simulink model "model"  (R2024a)
settings: Solver=FixedStepDiscrete  StartTime=0.0  StopTime=inf  FixedStep=0.01  RelTol=1e-3
libraries: simulink x1, spsMonostableLib x1
settings Model: Creator=Gabriel  LastModifiedBy=Gabriel

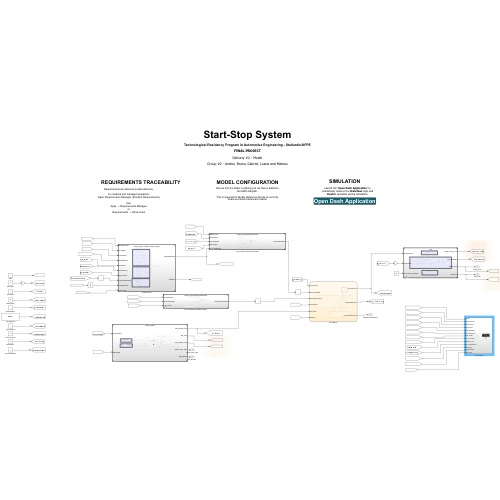
[thumbnail: Simulink's stored preview of the top-level diagram]
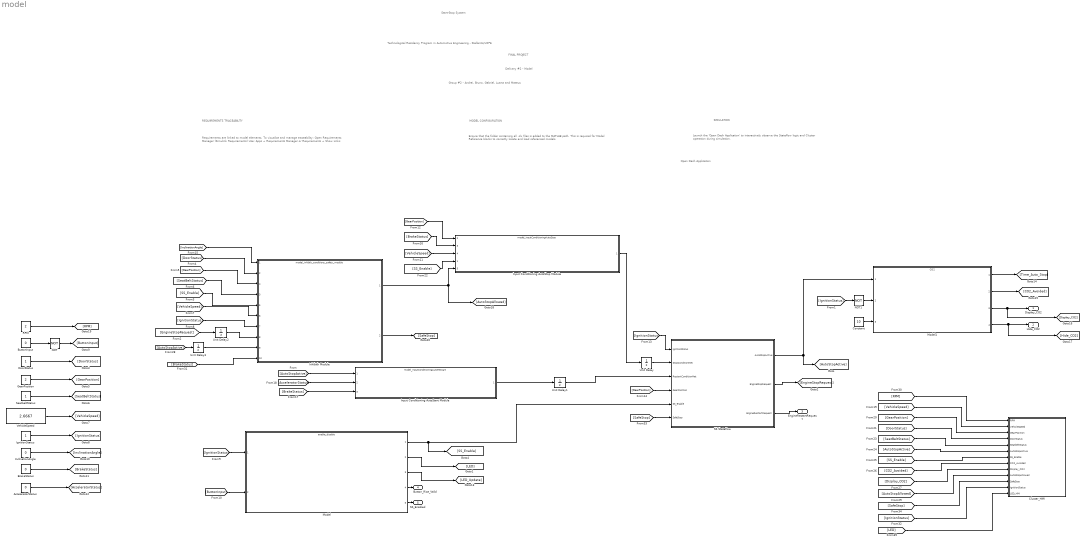
== system model ==
  note: Open Dash Application
  note: Technological Residency Program in Automotive Engineering - Stellantis/UFPE
  note: Start-Stop System
  note: FINAL PROJECT
  note: Group #2 - Andrei, Bruno, Gabriel, Luana and Mateus
  note: Delivery #2 - Model
  note: SIMULATION
  note: Launch the 'Open Dash Application' to interactively observe the Stateflow logic and Cluster operation during simulation.
  note: REQUIREMENTS TRACEABILITY
  note: Requirements are linked to model elements.
      |
      | To visualize and manage traceability:
      | Open Requirements Manager (Simulink Requirements)
      |
      | Use:
      | Apps → Requirements Manager
      | or
      | Requirements → Show Links
  note: Ensure that the folder containing all .slx files is added to the MATLAB path.
      |
      | This is required for Model Reference blocks to correctly locate and load referenced models.
  note: MODEL CONFIGURATION
  AcceleratorStatus : Constant  Value=0  OutDataTypeStr=boolean
  BrakeStatus : Constant  Value=0  OutDataTypeStr=boolean
  ButtonInput : Constant  Value=0  OutDataTypeStr=boolean
  Cluster_HMI : Subsystem
  Constant : Constant  Value=10
  DoorStatus : Constant  OutDataTypeStr=boolean
  GearPosition : Constant  Value=2
  IgnitionStatus : Constant  OutDataTypeStr=boolean
  InclinationAngle : Constant  Value=0
  Inhibith Module : ModelReference  ModelNameDialog=model_inhibth_conditions_safety_module.slx  SimulationMode=Normal  ModelReferenceVersion=1.14
      settings: PortSchema="{\"entries\":[{\"content\":{\"sides\":[{\"content\":{\"connectorIds\":[\"In1\",\"In2\",\"In4\",\"In3\",\"In5\",\"In6\",\"In7\",\"In8\",\"In9\",\"In10\"]},\"type\":\"ConnectorPlacement.EquallySpacedRectSide\",\"uuid\":\"a512ff0f-461c-49d9-bc5f-4a44ea731fcd\"},{\"content\":{\"connectorIds\":[\"Out1\",\"Out2\"],\"side\":\"RIGHT\"},\"type\":\"ConnectorPlacement.EquallySpacedRectSide\",\"uuid\":\"dd21159c-a948-4930-9666-9ab055a1217b\"},{\"content\":{\"side\":\"TOP\"},\"type\":\"ConnectorPlacement.EquallySpacedRectSide\",\"uuid\":\"5fbace01-0719-444d-b3d5-e5ff8fee5818\"}]},\"type\":\"ConnectorPlacement.EquallySpacedConnector\",\"uuid\":\"8aa1a26c-b679-4000-86cf-02a9aefd3465\"}],\"packageUris\":[\"http://schema.mathworks.com/mf0/Connector/R2020b\"],\"version\":\"1.0\"}"
  Input Conditioning AutoStart Module : ModelReference  ModelNameDialog=model_InputConditioningAutoRestart.slx  SimulationMode=Normal  ModelReferenceVersion=1.4
  Input Conditioning AutoStop Module : ModelReference  ModelNameDialog=model_InputConditioningAutoStop.slx  SimulationMode=Normal  ModelReferenceVersion=1.3
      settings: PortSchema="{\"entries\":[{\"content\":{\"sides\":[{\"content\":{\"connectorIds\":[\"In2\",\"In3\",\"In4\",\"In1\",\"In5\"]},\"type\":\"ConnectorPlacement.EquallySpacedRectSide\",\"uuid\":\"29c3241d-e620-43bc-b743-f10bc23ddf60\"},{\"content\":{\"connectorIds\":[\"Out1\"],\"side\":\"RIGHT\"},\"type\":\"ConnectorPlacement.EquallySpacedRectSide\",\"uuid\":\"375d0eb8-ed3e-4526-97ff-5015cdbb11d3\"},{\"content\":{\"side\":\"TOP\"},\"type\":\"ConnectorPlacement.EquallySpacedRectSide\",\"uuid\":\"7b1c3b74-98cc-495e-b24f-b127ed442c80\"}]},\"type\":\"ConnectorPlacement.EquallySpacedConnector\",\"uuid\":\"61a58fc7-57e7-4afa-ac3e-93f97ba24758\"}],\"packageUris\":[\"http://schema.mathworks.com/mf0/Connector/R2020b\"],\"version\":\"1.0\"}"
  Model : ModelReference  ModelNameDialog=enable_disable.slx  SimulationMode=Normal  ModelReferenceVersion=1.8
  Model1 : ModelReference  ModelNameDialog=CO2.slx  SimulationMode=Normal  ModelReferenceVersion=1.5
  NOT : Logic  Operator=NOT  IconShape=distinctive  AllPortsSameDT=off  OutDataTypeStr=boolean
  NOT1 : Logic  Operator=NOT  IconShape=distinctive  AllPortsSameDT=off  OutDataTypeStr=boolean
  RPM : Constant  Value=2  OutDataTypeStr=int8
  SS Stateflow : Stateflow chart  TreatAsAtomicUnit=on
  SeatbeltStatus : Constant  OutDataTypeStr=boolean
  Unit Delay : UnitDelay  SampleTime=-1  HasFrameUpgradeWarning=on
  Unit Delay1 : UnitDelay  SampleTime=-1  HasFrameUpgradeWarning=on
  Unit Delay2 : UnitDelay  SampleTime=0.1  HasFrameUpgradeWarning=on
  Unit Delay3 : UnitDelay  SampleTime=0.1  HasFrameUpgradeWarning=on
  VehicleSpeed : Constant  Value=2.6667
  Display_CO2 : Outport
  Hide_CO2 : Outport  Port=2
  EngineRestartRequest : Outport  Port=3
  Button_Rise_Valid : Outport  Port=4
  SS_Enabled : Outport  Port=5
  wires:
  DoorStatus/1 -> [DoorStatus]
  GearPosition/1 -> [GearPosition]
  SeatbeltStatus/1 -> [SeatBeltStatus]
  VehicleSpeed/1 -> [VehicleSpeed]
  IgnitionStatus/1 -> [IgnitionStatus]
  ButtonInput/1 -> NOT/1
  NOT/1 -> [ButtonInput]
  InclinationAngle/1 -> [InclinationAngle]
  BrakeStatus/1 -> [BrakeStatus]
  AcceleratorStatus/1 -> [AcceleratorStatus]
  Input Conditioning AutoStop Module/1 -> Unit Delay/1
  [GearPosition] -> Inhibith Module/4
  NOT1/1 -> Model1/2
  Model1/1 -> [Time_Auto_Stop]
  SS Stateflow/3(EngineRestartRequest) -> EngineRestartRequest/1
  [BrakeStatus] -> Input Conditioning AutoStart Module/3
  [VehicleSpeed] -> Input Conditioning AutoStop Module/4
  Model1/4 -> [Hide_CO2], Hide_CO2/1
  [GearPosition] -> Input Conditioning AutoStop Module/2
  Model1/3 -> [Display_CO2], Display_CO2/1
  [SS_Enable] -> Input Conditioning AutoStop Module/1
  Model/3 -> [LED_Update]
  Input Conditioning AutoStart Module/1 -> Unit Delay1/1
  Constant/1 -> Model1/3
  [InclinationAngle] -> Inhibith Module/1
  [IgnitionStatus] -> NOT1/1
  [IgnitionStatus] -> Model/1
  Model1/2 -> [CO2_Avoided]
  [GearPosition] -> SS Stateflow/4(GearPosition)
  Model/2 -> [LED]
  [ButtonInput] -> Model/2
  SS Stateflow/2(EngineStopRequest) -> [EngineStopRequest]
  [SeatBeltStatus] -> Inhibith Module/3
  [EngineStopRequest] -> Unit Delay2/1
  SS Stateflow/1(AutoStopActive) -> Model1/1, [AutoStopActive]
  Unit Delay1/1 -> SS Stateflow/3(RestartConditionMet)
  [IgnitionStatus] -> SS Stateflow/1(IgnitionStatus)
  Model/4 -> Button_Rise_Valid/1
  Inhibith Module/1 -> Input Conditioning AutoStop Module/5, [AutoStopAllowed]
  [VehicleSpeed] -> Inhibith Module/6
  [AcceleratorStatus] -> Input Conditioning AutoStart Module/2
  Unit Delay/1 -> SS Stateflow/2(StopConditionMet)
  [BrakeStatus] -> Input Conditioning AutoStop Module/3
  [DoorStatus] -> Inhibith Module/2
  [AutoStopActive] -> Input Conditioning AutoStart Module/1
  Model/5 -> SS_Enabled/1
  [SS_Enable] -> Inhibith Module/5
  [IgnitionStatus] -> Inhibith Module/7
  [VehicleSpeed] -> Cluster_HMI/2(VehicleSpeed)
  [GearPosition] -> Cluster_HMI/3(GearPosition)
  [DoorStatus] -> Cluster_HMI/4(DoorStatus)
  [SeatBeltStatus] -> Cluster_HMI/5(SeatbeltStatus)
  [AutoStopActive] -> Cluster_HMI/6(AutoStopActive)
  [CO2_Avoided] -> Cluster_HMI/8(CO2_Avoided)
  [Display_CO2] -> Cluster_HMI/9(Display_CO2)
  Model/1 -> [SS_Enable], SS Stateflow/5(SS_Enable)
  [SS_Enable] -> Cluster_HMI/7(SS_Enable)
  [AutoStopAllowed] -> Cluster_HMI/10(AutoStopAllowed)
  [RPM] -> Cluster_HMI/1(RPM)
  RPM/1 -> [RPM]
  [AutoStopActive] -> Unit Delay3/1
  [BrakeStatus] -> Inhibith Module/10
  Inhibith Module/2 -> [SafeStop]
  [SafeStop] -> SS Stateflow/6(SafeStop)
  [SafeStop] -> Cluster_HMI/11(SafeStop)
  Unit Delay2/1 -> Inhibith Module/8
  Unit Delay3/1 -> Inhibith Module/9
  [IgnitionStatus] -> Cluster_HMI/12(IgnitionStatus)
  [LED] -> Cluster_HMI/13(LED_HMI)

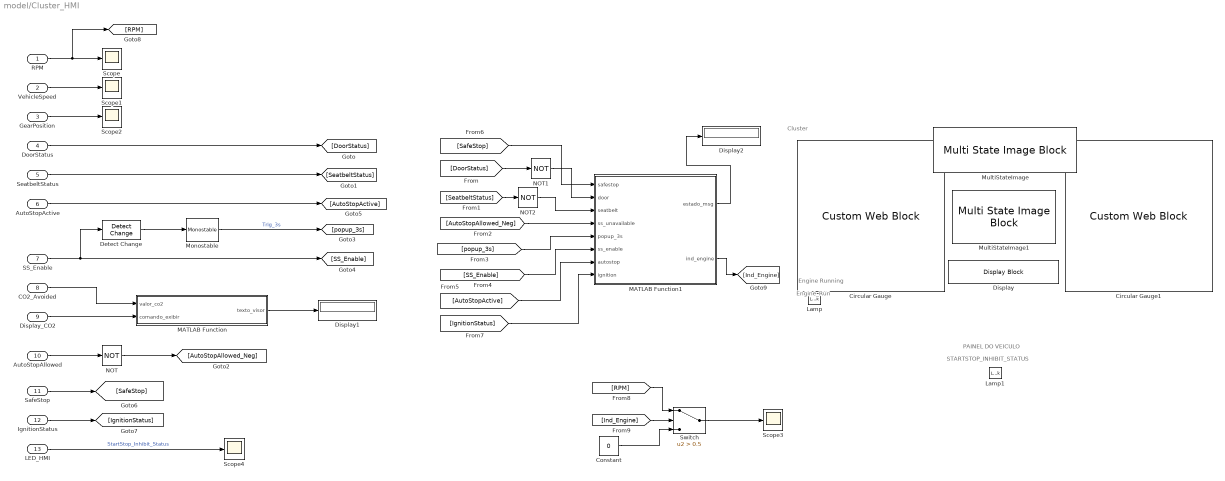
== system model/Cluster_HMI ==
  note: Engine_Run
  note: Engine Running
  note: Cluster
  note: PAINEL DO VEICULO
  note: STARTSTOP_INHIBIT_STATUS
  RPM : Inport
  VehicleSpeed : Inport  Port=2
  GearPosition : Inport  Port=3
  DoorStatus : Inport  Port=4
  SeatbeltStatus : Inport  Port=5
  AutoStopActive : Inport  Port=6
  SS_Enable : Inport  Port=7
  CO2_Avoided : Inport  Port=8
  Display_CO2 : Inport  Port=9
  AutoStopAllowed : Inport  Port=10
  SafeStop : Inport  Port=11
  IgnitionStatus : Inport  Port=12
  LED_HMI : Inport  Port=13
  Circular Gauge : CustomWebBlock  LabelPosition=Hide  ShowInitialText=on  Configuration="{\"components\":[{\"name\":\"CircularScaleComponent\",\"settings\":{\"bounds\":{\"max\":200,\"min\":0,\"tickInterval\":20},\"direction\":\"cw\",\"flipLimits\":0,\"innerRadius\":0.75,\"internalTickHeightScaleFactor\":1,\"labelColor\":[255,255,200],\"labelFont\":{\"font\":\"Arial\",\"fontSize\":12},\"labelRadius\":0.528,\"labelTransparency\":1,\"minorTickHeightScaleFactor\":0.2,\"needleImage\":{\"size\":[200,50],\"src\":\"data:image\\/svg+xml;base64,PD94bWwgdmVyc2lvbj0iMS4wIiBlbmNvZGluZz0idXRmLTgiPz4KPCEtLSBHZW5lcmF0b3I6IEFkb2JlIElsbHVzdHJhdG9yIDI0LjEuMiwgU1ZHIEV4cG9ydCBQbHVnLUluIC4gU1ZHIFZlcnNpb246IDYuMDAgQnVpbGQgMCkgIC0tPgo8c3ZnIHZlcnNpb249IjEuMSIgaWQ9IkxheWVyXzEiIHhtbG5zPSJodHRwOi8vd3d3LnczLm9yZy8yMDAwL3N2ZyIgeG1sbnM6eGxpbms9Imh0dHA6Ly93d3cudzMub3JnLzE5OTkveGxpbmsiIHg9IjBweCIgeT0iMHB4IgoJIHZpZXdCb3g9IjAgMCAyMDAgNTAiIHN0eWxlPSJlbmFibGUtYmFja2dyb3VuZDpuZXcgMCAwIDIwMCA1MDsiIHhtbDpzcGFjZT0icHJlc2VydmUiPgo8c3R5bGUgdHlwZT0idGV4dC9jc3MiPgoJLnN0MHtmaWxsOiNFQzIxMjc7fQo8L3N0eWxlPgo8cGF0aCBjbGFzcz0ic3QwIiBkPSJNMTYyLjgsMTMuN0MxNjksNC40LDE4MS43LDEuOSwxOTEsOC4xczExLjgsMTguOSw1LjYsMjguMnMtMTguOSwxMS44LTI4LjIsNS42bDAsMAoJQzE1OS4xLDM1LjYsMTU2LjYsMjMsMTYyLjgsMTMuN0wxNjIuOCwxMy43eiBNMTY1LjgsMTUuOGMtNS4xLDcuNi0zLjEsMTcuOSw0LjYsMjNjNy42LDUuMSwxNy45LDMuMSwyMy00LjYKCWM1LjEtNy42LDMuMS0xNy45LTQuNi0yM2wwLDBDMTgxLjIsNi4yLDE3MC45LDguMiwxNjUuOCwxNS44eiIvPgo8cGF0aCBjbGFzcz0ic3QwIiBkPSJNMC40LDI1Ljl2LTMuM2wxNTktMi41Yy0wLjcsMi42LTAuNyw1LjIsMCw3LjhMMC40LDI1Ljl6Ii8+CjxjaXJjbGUgY2xhc3M9InN0MCIgY3g9IjE3OS42IiBjeT0iMjQiIHI9IjAuNyIvPgo8L3N2Zz4K\"},\"needleOffset\":[0.18464878250906522,0],\"needleOrientation\":-45,\"needleRotation\":180,\"needleSize\":{\"height\":0.11741692305346914,\"width\":0.46108337545091255},\"outerRadius\":0.9,\"position\":[0.05,0.05,0.9,0.9],\"referencePoint\":\"auto\",\"scaleAngle\":270,\"scaleAngleOffset\":135,\"scaleColors\":[],\"scaleColorsSize\":0.2,\"scaleDirection\":\"CW\",\"scalePosition\":[0,0,1,1],\"showLabels\":1,\"showMinorTicks\":1,\"showSpanLine\":1,\"showTicks\":1,\"tickColor\":[252,252,197],\"tickTransparency\":1,\"valueBarColor\":[0,114,189],\"valueBarPosition\":[0,0,1,1],\"valueBarSize\":0.2,\"valueBarTransparency\":1}},{\"name\":\"BackgroundImageComponent\",\"settings\":{\"image\":{\"size\":[500,500],\"src\":\"data:image\\/svg+xml;base64,PD94bWwgdmVyc2lvbj0iMS4wIiBlbmNvZGluZz0iVVRGLTgiIHN0YW5kYWxvbmU9Im5vIj8+CjxzdmcKICAgeG1sbnM6ZGM9Imh0dHA6Ly9wdXJsLm9yZy9kYy9lbGVtZW50cy8xLjEvIgogICB4bWxuczpjYz0iaHR0cDovL2NyZWF0aXZlY29tbW9ucy5vcmcvbnMjIgogICB4bWxuczpyZGY9Imh0dHA6Ly93d3cudzMub3JnLzE5OTkvMDIvMjItcmRmLXN5bnRheC1ucyMiCiAgIHhtbG5zOnN2Zz0iaHR0cDovL3d3dy53My5vcmcvMjAwMC9zdmciCiAgIHhtbG5zPSJodHRwOi8vd3d3LnczLm9yZy8yMDAwL3N2ZyIKICAgeG1sbnM6 ...(+9964 chars)\"},\"position\":[0,0,1,1],\"scaleMode\":\"0\"}},{\"name\":\"ForegroundImageComponent\",\"settings\":{\"image\":{\"size\":[0,0],\"src\":\"default\",\"srcOrientation\":[]},\"isForeground\":1,\"position\":[0,0,1,1],\"scaleMode\":\"0\"}}],\"settings\":{\"BindingType\":\"signal\",\"aspectRatio\":1.032258064516129,\"backgroundColor\":[0,0,0,\"1\"],\"backgroundOffset\":1,\"backgroundOpacity\":1,\"direction\":\"cw\",\"fixedAspectRatio\":\"on\",\"flipLimits\":0,\"orientation\":\"horizontal\",\"showBackgroundColor\":false,\"value\":0,\"version\":\"R2023a\"},\"type\":\"CircularGauge\"}"
  Circular Gauge1 : CustomWebBlock  LabelPosition=Hide  ShowInitialText=on  Configuration="{\"components\":[{\"name\":\"CircularScaleComponent\",\"settings\":{\"bounds\":{\"max\":8,\"min\":0,\"tickInterval\":1},\"direction\":\"cw\",\"flipLimits\":0,\"innerRadius\":0.75,\"internalTickHeightScaleFactor\":1,\"labelColor\":[255,255,200],\"labelFont\":{\"font\":\"Arial\",\"fontSize\":12},\"labelRadius\":0.528,\"labelTransparency\":1,\"minorTickHeightScaleFactor\":0.2,\"needleImage\":{\"size\":[200,50],\"src\":\"data:image\\/svg+xml;base64,PD94bWwgdmVyc2lvbj0iMS4wIiBlbmNvZGluZz0idXRmLTgiPz4KPCEtLSBHZW5lcmF0b3I6IEFkb2JlIElsbHVzdHJhdG9yIDI0LjEuMiwgU1ZHIEV4cG9ydCBQbHVnLUluIC4gU1ZHIFZlcnNpb246IDYuMDAgQnVpbGQgMCkgIC0tPgo8c3ZnIHZlcnNpb249IjEuMSIgaWQ9IkxheWVyXzEiIHhtbG5zPSJodHRwOi8vd3d3LnczLm9yZy8yMDAwL3N2ZyIgeG1sbnM6eGxpbms9Imh0dHA6Ly93d3cudzMub3JnLzE5OTkveGxpbmsiIHg9IjBweCIgeT0iMHB4IgoJIHZpZXdCb3g9IjAgMCAyMDAgNTAiIHN0eWxlPSJlbmFibGUtYmFja2dyb3VuZDpuZXcgMCAwIDIwMCA1MDsiIHhtbDpzcGFjZT0icHJlc2VydmUiPgo8c3R5bGUgdHlwZT0idGV4dC9jc3MiPgoJLnN0MHtmaWxsOiNFQzIxMjc7fQo8L3N0eWxlPgo8cGF0aCBjbGFzcz0ic3QwIiBkPSJNMTYyLjgsMTMuN0MxNjksNC40LDE4MS43LDEuOSwxOTEsOC4xczExLjgsMTguOSw1LjYsMjguMnMtMTguOSwxMS44LTI4LjIsNS42bDAsMAoJQzE1OS4xLDM1LjYsMTU2LjYsMjMsMTYyLjgsMTMuN0wxNjIuOCwxMy43eiBNMTY1LjgsMTUuOGMtNS4xLDcuNi0zLjEsMTcuOSw0LjYsMjNjNy42LDUuMSwxNy45LDMuMSwyMy00LjYKCWM1LjEtNy42LDMuMS0xNy45LTQuNi0yM2wwLDBDMTgxLjIsNi4yLDE3MC45LDguMiwxNjUuOCwxNS44eiIvPgo8cGF0aCBjbGFzcz0ic3QwIiBkPSJNMC40LDI1Ljl2LTMuM2wxNTktMi41Yy0wLjcsMi42LTAuNyw1LjIsMCw3LjhMMC40LDI1Ljl6Ii8+CjxjaXJjbGUgY2xhc3M9InN0MCIgY3g9IjE3OS42IiBjeT0iMjQiIHI9IjAuNyIvPgo8L3N2Zz4K\"},\"needleOffset\":[0.18464878250906522,0],\"needleOrientation\":-45,\"needleRotation\":180,\"needleSize\":{\"height\":0.11741692305346914,\"width\":0.46108337545091255},\"outerRadius\":0.9,\"position\":[0.05,0.05,0.9,0.9],\"referencePoint\":\"auto\",\"scaleAngle\":270,\"scaleAngleOffset\":135,\"scaleColors\":[],\"scaleColorsSize\":0.2,\"scaleDirection\":\"CW\",\"scalePosition\":[0,0,1,1],\"showLabels\":1,\"showMinorTicks\":1,\"showSpanLine\":1,\"showTicks\":1,\"tickColor\":[252,252,197],\"tickTransparency\":1,\"valueBarColor\":[0,114,189],\"valueBarPosition\":[0,0,1,1],\"valueBarSize\":0.2,\"valueBarTransparency\":1}},{\"name\":\"BackgroundImageComponent\",\"settings\":{\"image\":{\"size\":[500,500],\"src\":\"data:image\\/svg+xml;base64,PD94bWwgdmVyc2lvbj0iMS4wIiBlbmNvZGluZz0iVVRGLTgiIHN0YW5kYWxvbmU9Im5vIj8+CjxzdmcKICAgeG1sbnM6ZGM9Imh0dHA6Ly9wdXJsLm9yZy9kYy9lbGVtZW50cy8xLjEvIgogICB4bWxuczpjYz0iaHR0cDovL2NyZWF0aXZlY29tbW9ucy5vcmcvbnMjIgogICB4bWxuczpyZGY9Imh0dHA6Ly93d3cudzMub3JnLzE5OTkvMDIvMjItcmRmLXN5bnRheC1ucyMiCiAgIHhtbG5zOnN2Zz0iaHR0cDovL3d3dy53My5vcmcvMjAwMC9zdmciCiAgIHhtbG5zPSJodHRwOi8vd3d3LnczLm9yZy8yMDAwL3N2ZyIKICAgeG1sbnM6 ...(+9964 chars)\"},\"position\":[0,0,1,1],\"scaleMode\":\"0\"}},{\"name\":\"ForegroundImageComponent\",\"settings\":{\"image\":{\"size\":[0,0],\"src\":\"default\",\"srcOrientation\":[]},\"isForeground\":1,\"position\":[0,0,1,1],\"scaleMode\":\"0\"}}],\"settings\":{\"BindingType\":\"signal\",\"aspectRatio\":1.032258064516129,\"backgroundColor\":[0,0,0,\"1\"],\"backgroundOffset\":1,\"backgroundOpacity\":1,\"direction\":\"cw\",\"fixedAspectRatio\":\"on\",\"flipLimits\":0,\"orientation\":\"horizontal\",\"showBackgroundColor\":false,\"value\":0,\"version\":\"R2023a\"},\"type\":\"CircularGauge\"}"
  Constant : Constant  Value=0
  Detect Change : simulink/Logic and Bit Operations/Detect Change  vinit=0  OutDataTypeStr=boolean
  Display : DisplayBlock  LabelPosition=Hide  Transparency=1
  Display1 : Display
  Display2 : Display
  Lamp : LampBlock  LabelPosition=Hide
  Lamp1 : LampBlock  LabelPosition=Hide
  MATLAB Function : MATLAB Function  TreatAsAtomicUnit=on
  MATLAB Function1 : MATLAB Function  TreatAsAtomicUnit=on
  Monostable : spsMonostableLib/Monostable  EdgeDetect=Rising  PulseDuration=3  ic=0  Ts=0
      settings: LibrarySourceBlock=sps_lib/Control/Monostable
  MultiStateImage : MultiStateImageBlock  LabelPosition=Hide
  MultiStateImage1 : MultiStateImageBlock  LabelPosition=Hide
  NOT : Logic  Operator=NOT  IconShape=distinctive  AllPortsSameDT=off  OutDataTypeStr=boolean
  NOT1 : Logic  Operator=NOT  IconShape=distinctive  AllPortsSameDT=off  OutDataTypeStr=boolean
  NOT2 : Logic  Operator=NOT  IconShape=distinctive  AllPortsSameDT=off  OutDataTypeStr=boolean
  Scope{,1..4} (5 alike) : Scope
  Switch : Switch  Criteria=u2 > Threshold  Threshold=0.5  SaturateOnIntegerOverflow=off  InputSameDT=off
  wires:
  SS_Enable/1 -> Detect Change/1, [SS_Enable]
  VehicleSpeed/1 -> Scope1/1
  GearPosition/1 -> Scope2/1
  CO2_Avoided/1 -> MATLAB Function/1(valor_co2)
  Display_CO2/1 -> MATLAB Function/2(comando_exibir)
  Detect Change/1 -> Monostable/1
  [DoorStatus] -> NOT1/1
  [SeatbeltStatus] -> NOT2/1
  [AutoStopAllowed_Neg] -> MATLAB Function1/4(ss_unavailable)
  [popup_3s] -> MATLAB Function1/5(popup_3s)
  [SS_Enable] -> MATLAB Function1/6(ss_enable)
  DoorStatus/1 -> [DoorStatus]
  SeatbeltStatus/1 -> [SeatbeltStatus]
  AutoStopAllowed/1 -> NOT/1
  NOT/1 -> [AutoStopAllowed_Neg]
  Monostable/1 -> [popup_3s]  "Trig_3s"
  AutoStopActive/1 -> [AutoStopActive]
  NOT1/1 -> MATLAB Function1/2(door)
  NOT2/1 -> MATLAB Function1/3(seatbelt)
  [AutoStopActive] -> MATLAB Function1/7(autostop)
  RPM/1 -> [RPM], Scope/1
  MATLAB Function/1(texto_visor) -> Display1/1
  MATLAB Function1/1(estado_msg) -> Display2/1
  [SafeStop] -> MATLAB Function1/1(safestop)
  SafeStop/1 -> [SafeStop]
  IgnitionStatus/1 -> [IgnitionStatus]
  MATLAB Function1/2(ind_engine) -> [Ind_Engine]
  [IgnitionStatus] -> MATLAB Function1/8(ignition)
  [RPM] -> Switch/1
  [Ind_Engine] -> Switch/2
  Constant/1 -> Switch/3
  Switch/1 -> Scope3/1
  LED_HMI/1 -> Scope4/1  "StartStop_Inhibit_Status"

== matlab function model/Cluster_HMI/MATLAB Function1 ==
  data: safestop input; door input; estado_msg output; seatbelt input; ss_unavailable input; popup_3s input; ss_enable input; autostop input; ignition input; ind_engine output
function [estado_msg, ind_engine] = arbitro_hmi(safestop, door, seatbelt, ss_unavailable, popup_3s, ss_enable, autostop, ignition)
    
    % --- LÓGICA DO LAMP (Motor Running vs Off) ---
    % O motor só está rodando (1) se a ignição estiver ligada, 
    % e o sistema não tiver desligado o motor (autostop ou safestop).
    if (ignition == 1) && (autostop == 0) && (safestop == 0)
        ind_engine = 1; % Motor Ligado (Lamp ON)
    else
        ind_engine = 0; % Motor Desligado (Lamp OFF)
    end

    % --- LÓGICA DO CLUSTER CENTRAL (Mensagens) ---
    estado_msg = 0; % Tela Limpa
    
    % PRIORIDADE ZERO: Bloqueio de Segurança (Safe Stop)
    if safestop == 1
        estado_msg = 7; 
        
    % PRIORIDADE 1: Falhas e Segurança (Crítico)
    elseif door == 1
        estado_msg = 1; 
        
    elseif seatbelt == 1 
        estado_msg = 2; 
        
    % PRIORIDADE 2: Pop-up Temporário
    elseif popup_3s == 1
        if ss_enable == 1
            estado_msg = 4; 
        else
            estado_msg = 5; 
        end
        
    % PRIORIDADE 3: Operação Normal (AutoStop)
    elseif autostop == 1
        estado_msg = 6; 
        
    % PRIORIDADE 4: Sistema Indisponível (Laranja)
    elseif ss_unavailable == 1 && autostop == 0 && ss_enable == 1
        estado_msg = 3; 
    end
end

== matlab function model/Cluster_HMI/MATLAB Function ==
  data: valor_co2 input; texto_visor output; comando_exibir input
function texto_visor = logica_co2(valor_co2, comando_exibir)
    % O Simulink exige que o número seja inteiro (round) para virar string
    if comando_exibir == 1
        texto_visor = string(round(valor_co2)) + " g CO2 Evitado";
    else
        texto_visor = ""; 
    end
end

== stateflow chart model/SS Stateflow ==
  state VehicleOff
    entry:
    AutoStopActive =  false;
    EngineStopRequest = false;
    EngineRestartRequest =  false;
  state SS_Available
    state EngineRunning
      entry:
      AutoStopActive = false;
      EngineStopRequest = false;
    state AutoStopActive
      entry:
      AutoStopActive = true;
      EngineRestartRequest = false;
    (default) -> EngineRunning
    AutoStopActive -> EngineRunning : [(RestartConditionMet || GearPosition ~= 2 || after(180, sec)) && SafeStop == 0]{EngineRestartRequest = true;}
    EngineRunning -> AutoStopActive : [StopConditionMet]{EngineStopRequest = true;}
  state SS_Unavailable
    entry:
    AutoStopActive = false;
    EngineStopRequest = false;
    EngineRestartRequest = false;
  (default) -> VehicleOff
  SS_Available -> VehicleOff [order 2] : [IgnitionStatus == false]
  VehicleOff -> SS_Available : [IgnitionStatus == true]
  SS_Available -> SS_Unavailable [order 1] : [SS_Enable == false]
  SS_Unavailable -> SS_Available : [SS_Enable == true]
  data: IgnitionStatus input boolean; StopConditionMet input; AutoStopActive output boolean; RestartConditionMet input; EngineStopRequest output; EngineRestartRequest output; GearPosition input; SS_Enable input; SafeStop input
